simulink model "e3"  (R2022b)
settings: Solver=VariableStepAuto  StartTime=0.0  StopTime=40  RelTol=1e-3
settings Model: Creator=bn19b  LastModifiedBy=bn19b

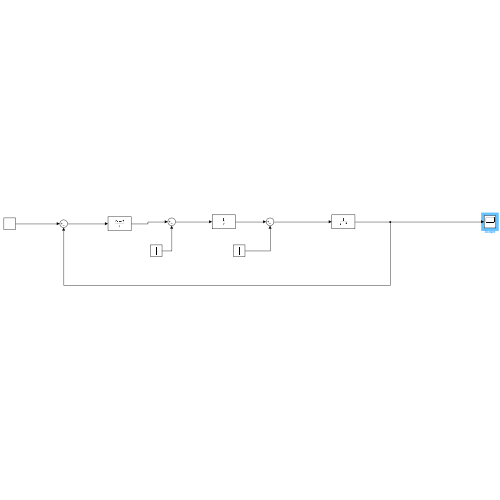
[thumbnail: Simulink's stored preview of the top-level diagram]
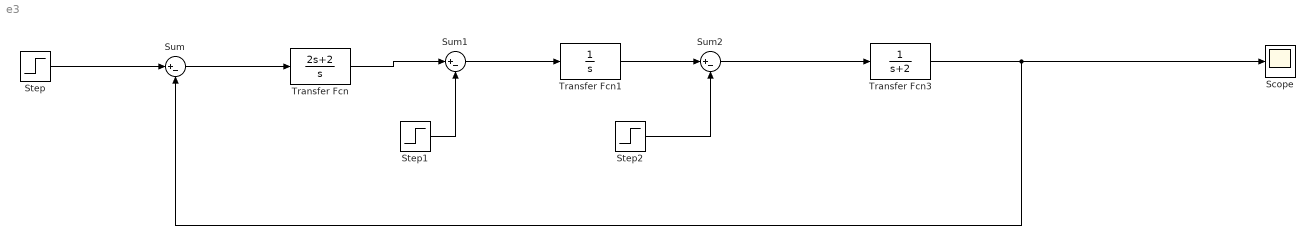
== system e3 ==
  Scope : Scope
  Step : Step  SampleTime=0
  Step1 : Step  Time=7  After=0.3  SampleTime=0
  Step2 : Step  Time=15  After=0.4  SampleTime=0
  Sum : Sum  Inputs=|+-
  Sum1 : Sum  Inputs=|+-
  Sum2 : Sum  Inputs=|+-
  Transfer Fcn : TransferFcn  Numerator=[2 2]  Denominator=[1 0]
  Transfer Fcn1 : TransferFcn  Denominator=[1 0]
  Transfer Fcn3 : TransferFcn  Denominator=[1 2]
  wires:
  Step/1 -> Sum/1
  Transfer Fcn/1 -> Sum1/1
  Step1/1 -> Sum1/2
  Sum1/1 -> Transfer Fcn1/1
  Sum/1 -> Transfer Fcn/1
  Transfer Fcn1/1 -> Sum2/1
  Step2/1 -> Sum2/2
  Sum2/1 -> Transfer Fcn3/1
  Transfer Fcn3/1 -> Scope/1, Sum/2
